simulink model "robust_tracking_integral"  (R2020b)
settings: Solver=ode45  StartTime=0.0  StopTime=5  FixedStep=T/10  RelTol=1e-3
values from neighbouring files (symbols this model uses):
  daq =     [params_inertial_case.mat]    (also in params_resonant_case.mat)
  degs2rpm = 0.166666666667    [params_inertial_case.mat]    (also in params_resonant_case.mat)
  drv =     [params_inertial_case.mat]    (also in params_resonant_case.mat)
  gbox =     [params_inertial_case.mat]    (also in params_resonant_case.mat)
  mld =     [params_inertial_case.mat]    (also in params_resonant_case.mat)
  mot =     [params_inertial_case.mat]    (also in params_resonant_case.mat)
  rads2rpm = 9.54929658551    [params_inertial_case.mat]    (also in params_resonant_case.mat)
  rpm2rads = 0.10471975512    [params_inertial_case.mat]    (also in params_resonant_case.mat)
  sens =     [params_inertial_case.mat]    (also in params_resonant_case.mat)
  tau_hat = 0.00714370660323    [params_estimated_LAB0.mat]
undefined symbols (not defined in the file or in its folder): Beq, ctrl, denH1, Jeq, k_spring, Ke, Ki, N_u, N_x, numH1, step_size
settings Model: Creator=utente  LastModifiedBy=gioel
settings DataIOCC: ReturnWorkspaceOutputs=off

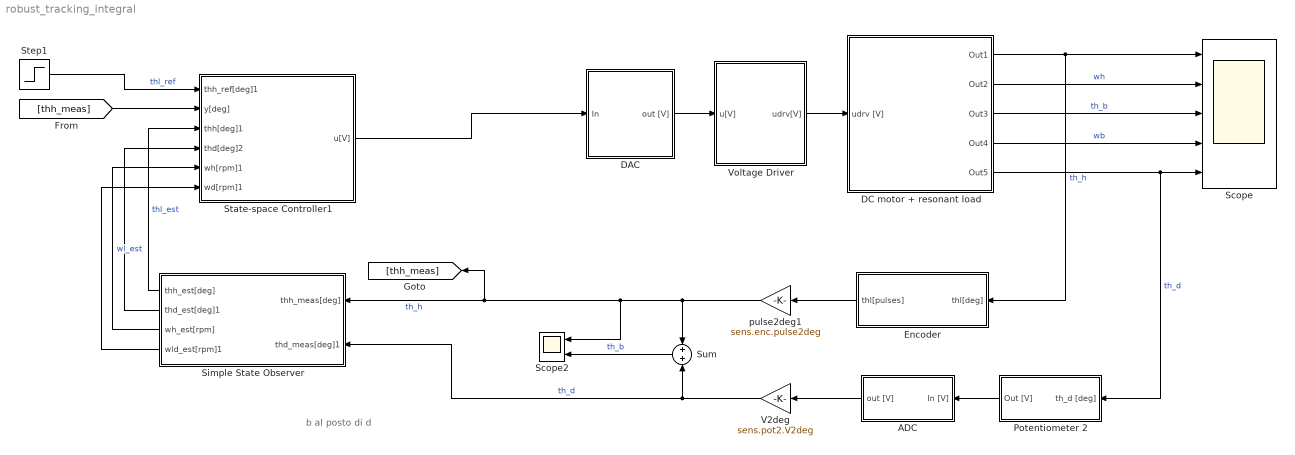
== system robust_tracking_integral ==
  note: b al posto di d
  ADC : Subsystem
  DAC : Subsystem
  DC motor + resonant load : Subsystem
  Encoder : Subsystem
  Potentiometer 2 : Subsystem
  Scope : Scope  NumInputPorts=5
  Scope2 : Scope  NumInputPorts=2
  Simple State Observer : Subsystem
  State-space Controller1 : Subsystem
  Step1 : Step  After=step_size  SampleTime=0
  Sum : Sum
  V2deg : Gain  Gain=sens.pot2.V2deg
  Voltage Driver : Subsystem
  pulse2deg1 : Gain  Gain=sens.enc.pulse2deg
  wires:
  DC motor + resonant load/3(Out3) -> Scope/3  "th_b"
  DAC/1(out [V]) -> Voltage Driver/1(u[V])
  DC motor + resonant load/2(Out2) -> Scope/2  "wh"
  DC motor + resonant load/1(Out1) -> Scope/1, Encoder/1(thl[deg])  "th_h"
  DC motor + resonant load/5(Out5) -> Scope/5, Potentiometer 2/1(th_d [deg])  "th_d"
  Encoder/1(thl[pulses]) -> pulse2deg1/1
  Voltage Driver/1(udrv[V]) -> DC motor + resonant load/1(udrv [V])
  pulse2deg1/1 -> Scope2/1, Simple State Observer/1(thh_meas[deg]), [thh_meas], Sum/1  "th_h"
  Potentiometer 2/1(Out [V]) -> ADC/1(In [V])
  V2deg/1 -> Simple State Observer/2(thd_meas[deg]1), Sum/2  "th_d"
  Sum/1 -> Scope2/2  "th_b"
  ADC/1(out [V]) -> V2deg/1
  DC motor + resonant load/4(Out4) -> Scope/4  "wb"
  Step1/1 -> State-space Controller1/1(thh_ref[deg]1)  "thl_ref"
  Simple State Observer/1(thh_est[deg]) -> State-space Controller1/3(thh[deg]1)  "thl_est"
  Simple State Observer/2(thd_est[deg]1) -> State-space Controller1/4(thd[deg]2)
  Simple State Observer/3(wh_est[rpm]) -> State-space Controller1/5(wh[rpm]1)  "wl_est"
  Simple State Observer/4(wld_est[rpm]1) -> State-space Controller1/6(wd[rpm]1)
  State-space Controller1/1(u[V]) -> DAC/1(In)
  [thh_meas] -> State-space Controller1/2(y[deg])

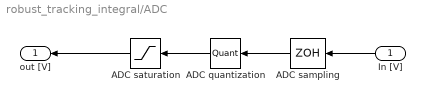
== system robust_tracking_integral/ADC ==
  In [V] : Inport
  ADC quantization : Quantizer  QuantizationInterval=daq.dac.q
  ADC saturation : Saturate  UpperLimit=daq.dac.fs  LowerLimit=-daq.dac.fs
  ADC sampling : ZeroOrderHold  SampleTime=0.001
  out [V] : Outport
  wires:
  ADC saturation/1 -> out [V]/1
  In [V]/1 -> ADC sampling/1
  ADC quantization/1 -> ADC saturation/1
  ADC sampling/1 -> ADC quantization/1

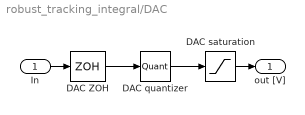
== system robust_tracking_integral/DAC ==
  In : Inport
  DAC quantizer : Quantizer  QuantizationInterval=daq.dac.q
  DAC saturation : Saturate  UpperLimit=daq.dac.fs  LowerLimit=-daq.dac.fs
  DAC ZOH : ZeroOrderHold  SampleTime=0.001
  out [V] : Outport
  wires:
  DAC ZOH/1 -> DAC quantizer/1
  DAC quantizer/1 -> DAC saturation/1
  In/1 -> DAC ZOH/1
  DAC saturation/1 -> out [V]/1

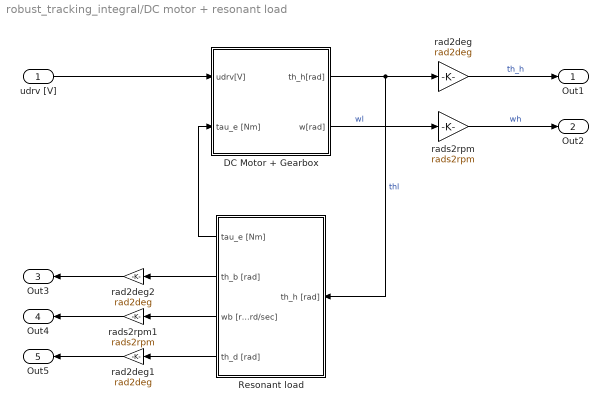
== system robust_tracking_integral/DC motor + resonant load ==
  udrv [V] : Inport
  DC Motor + Gearbox : Subsystem
  Resonant load : Subsystem
  rad2deg : Gain  Gain=rad2deg
  rad2deg1 : Gain  Gain=rad2deg
  rad2deg2 : Gain  Gain=rad2deg
  "rads2rpm " : Gain  Gain=rads2rpm
  "rads2rpm1 " : Gain  Gain=rads2rpm
  Out1 : Outport
  Out2 : Outport  Port=2
  Out3 : Outport  Port=3
  Out4 : Outport  Port=4
  Out5 : Outport  Port=5
  wires:
  Resonant load/3(wb [rard/sec]) -> "rads2rpm1 "/1
  Resonant load/4(th_d [rad]) -> rad2deg1/1
  "rads2rpm1 "/1 -> Out4/1
  rad2deg/1 -> Out1/1  "th_h"
  "rads2rpm "/1 -> Out2/1  "wh"
  rad2deg2/1 -> Out3/1
  udrv [V]/1 -> DC Motor + Gearbox/1(udrv[V])
  Resonant load/2(th_b [rad]) -> rad2deg2/1
  rad2deg1/1 -> Out5/1
  DC Motor + Gearbox/1(th_h[rad]) -> Resonant load/1(th_h [rad]), rad2deg/1  "thl"
  DC Motor + Gearbox/2(w[rad]) -> "rads2rpm "/1  "wl"
  Resonant load/1(tau_e [Nm]) -> DC Motor + Gearbox/2(tau_e [Nm])

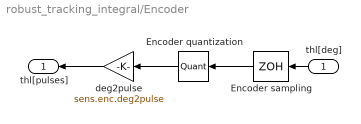
== system robust_tracking_integral/Encoder ==
  thl[deg] : Inport
  Encoder quantization : Quantizer  QuantizationInterval=sens.enc.pulse2deg
  Encoder sampling : ZeroOrderHold  SampleTime=-1
  deg2pulse : Gain  Gain=sens.enc.deg2pulse
  thl[pulses] : Outport
  wires:
  thl[deg]/1 -> Encoder sampling/1
  Encoder quantization/1 -> deg2pulse/1
  Encoder sampling/1 -> Encoder quantization/1
  deg2pulse/1 -> thl[pulses]/1

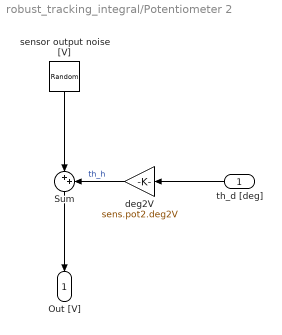
== system robust_tracking_integral/Potentiometer 2 ==
  th_d [deg] : Inport
  Sum : Sum  Inputs=|++
  deg2V : Gain  Gain=sens.pot2.deg2V
  "sensor output noise [V] " : RandomNumber  Variance=3.5e-7  SampleTime=0.1
  Out [V] : Outport
  wires:
  th_d [deg]/1 -> deg2V/1
  deg2V/1 -> Sum/2  "th_h"
  "sensor output noise [V] "/1 -> Sum/1
  Sum/1 -> Out [V]/1

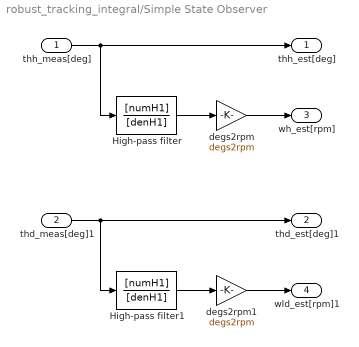
== system robust_tracking_integral/Simple State Observer ==
  thh_meas[deg] : Inport
  thd_meas[deg]1 : Inport  Port=2
  High-pass filter : TransferFcn  Numerator=[numH1]  Denominator=[denH1]
  High-pass filter1 : TransferFcn  Numerator=[numH1]  Denominator=[denH1]
  degs2rpm : Gain  Gain=degs2rpm
  degs2rpm1 : Gain  Gain=degs2rpm
  thh_est[deg] : Outport
  thd_est[deg]1 : Outport  Port=2
  wh_est[rpm] : Outport  Port=3
  wld_est[rpm]1 : Outport  Port=4
  wires:
  thh_meas[deg]/1 -> thh_est[deg]/1, High-pass filter/1
  High-pass filter/1 -> degs2rpm/1
  degs2rpm/1 -> wh_est[rpm]/1
  thd_meas[deg]1/1 -> thd_est[deg]1/1, High-pass filter1/1
  High-pass filter1/1 -> degs2rpm1/1
  degs2rpm1/1 -> wld_est[rpm]1/1

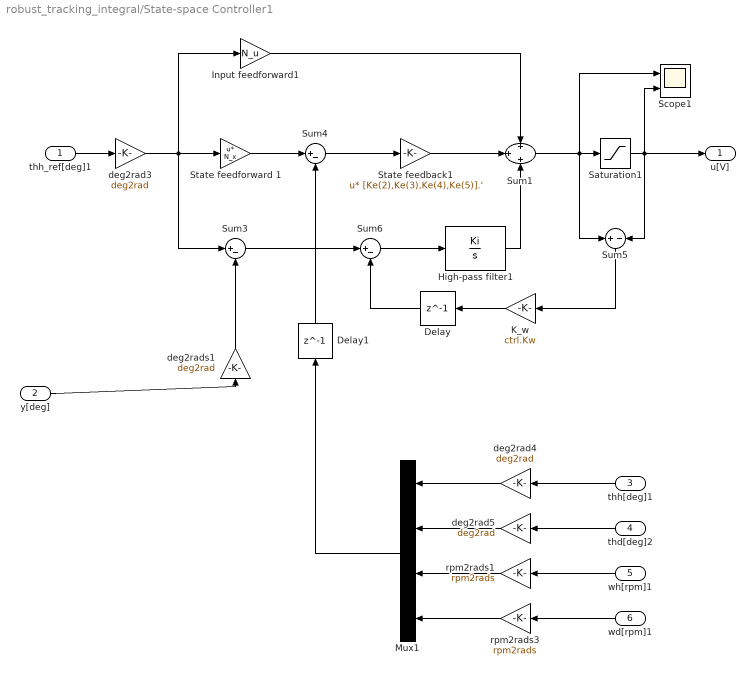
== system robust_tracking_integral/State-space Controller1 ==
  thh_ref[deg]1 : Inport
  y[deg] : Inport  Port=2
  thh[deg]1 : Inport  Port=3
  thd[deg]2 : Inport  Port=4
  wh[rpm]1 : Inport  Port=5
  wd[rpm]1 : Inport  Port=6
  Delay : Delay  DelayLength=1  InitialCondition=0
  Delay1 : Delay  DelayLength=1  InitialCondition=0
  High-pass filter1 : TransferFcn  Numerator=Ki  Denominator=[1 0]
  Input feedforward1 : Gain  Gain=N_u
  K_w : Gain  Gain=ctrl.Kw
  Mux1 : Mux
  Saturation1 : Saturate  UpperLimit=10  LowerLimit=-10
  Scope1 : Scope  NumInputPorts=2
  State feedback1 : Gain  Gain=[Ke(2),Ke(3),Ke(4),Ke(5)].'  Multiplication=Matrix(u*K)
  State feedforward	1 : Gain  Gain=N_x  Multiplication=Matrix(u*K)
  Sum1 : Sum  Inputs=+|+|+
  Sum3 : Sum  Inputs=|+-
  Sum4 : Sum  Inputs=|+-
  Sum5 : Sum  Inputs=+|-
  Sum6 : Sum  Inputs=|+-
  deg2rad3 : Gain  Gain=deg2rad
  deg2rad4 : Gain  Gain=deg2rad
  deg2rad5 : Gain  Gain=deg2rad
  deg2rads1 : Gain  Gain=deg2rad
  rpm2rads1 : Gain  Gain=rpm2rads
  rpm2rads3 : Gain  Gain=rpm2rads
  u[V] : Outport
  wires:
  Delay/1 -> Sum6/2
  Sum6/1 -> High-pass filter1/1
  deg2rads1/1 -> Sum3/2
  y[deg]/1 -> deg2rads1/1
  Sum1/1 -> Sum5/1, Scope1/1, Saturation1/1
  Delay1/1 -> Sum4/2
  K_w/1 -> Delay/1
  High-pass filter1/1 -> Sum1/3
  Sum5/1 -> K_w/1
  Sum3/1 -> Sum6/1
  State feedback1/1 -> Sum1/2
  Sum4/1 -> State feedback1/1
  deg2rad3/1 -> Sum3/1, Input feedforward1/1, State feedforward	1/1
  Saturation1/1 -> Sum5/2, Scope1/2, u[V]/1
  State feedforward	1/1 -> Sum4/1
  Input feedforward1/1 -> Sum1/1
  deg2rad5/1 -> Mux1/2
  Mux1/1 -> Delay1/1
  rpm2rads1/1 -> Mux1/3
  wd[rpm]1/1 -> rpm2rads3/1
  wh[rpm]1/1 -> rpm2rads1/1
  thh[deg]1/1 -> deg2rad4/1
  deg2rad4/1 -> Mux1/1
  thd[deg]2/1 -> deg2rad5/1
  rpm2rads3/1 -> Mux1/4
  thh_ref[deg]1/1 -> deg2rad3/1

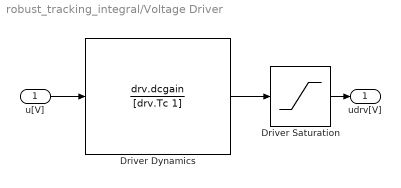
== system robust_tracking_integral/Voltage Driver ==
  u[V] : Inport
  Driver Dynamics : TransferFcn  Numerator=drv.dcgain  Denominator=[drv.Tc 1]
  Driver Saturation : Saturate  UpperLimit=12  LowerLimit=-12
  udrv[V] : Outport
  wires:
  Driver Dynamics/1 -> Driver Saturation/1
  Driver Saturation/1 -> udrv[V]/1
  u[V]/1 -> Driver Dynamics/1

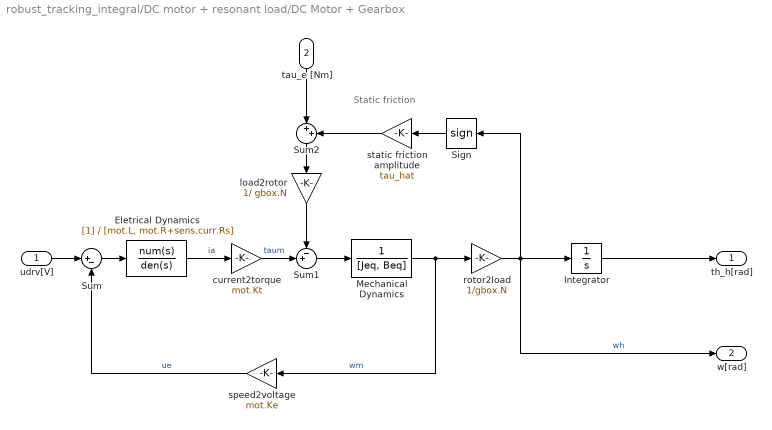
== system robust_tracking_integral/DC motor + resonant load/DC Motor + Gearbox ==
  note: Static friction
  udrv[V] : Inport
  tau_e [Nm] : Inport  Port=2
  Eletrical Dynamics : TransferFcn  Denominator=[mot.L, mot.R+sens.curr.Rs]
  Integrator : Integrator
  Mechanical Dynamics : TransferFcn  Denominator=[Jeq, Beq]
  Sign : Signum  ZeroCross=off
  Sum : Sum  Inputs=|+-
  Sum1 : Sum  Inputs=-+|
  Sum2 : Sum  Inputs=|++
  current2torque : Gain  Gain=mot.Kt
  load2rotor : Gain  Gain=1/ gbox.N
  rotor2load : Gain  Gain=1/gbox.N
  speed2voltage : Gain  Gain=mot.Ke
  static friction amplitude : Gain  Gain=tau_hat
  th_h[rad] : Outport  VectorParamsAs1DForOutWhenUnconnected=off
  w[rad] : Outport  Port=2  VectorParamsAs1DForOutWhenUnconnected=off
  wires:
  Eletrical Dynamics/1 -> current2torque/1  "ia"
  udrv[V]/1 -> Sum/1
  Sum/1 -> Eletrical Dynamics/1
  current2torque/1 -> Sum1/2  "taum"
  Sum1/1 -> Mechanical Dynamics/1
  Mechanical Dynamics/1 -> rotor2load/1, speed2voltage/1  "wm"
  rotor2load/1 -> w[rad]/1, Integrator/1, Sign/1  "wh"
  Integrator/1 -> th_h[rad]/1
  Sign/1 -> static friction amplitude/1
  speed2voltage/1 -> Sum/2  "ue"
  load2rotor/1 -> Sum1/1
  Sum2/1 -> load2rotor/1
  static friction amplitude/1 -> Sum2/2
  tau_e [Nm]/1 -> Sum2/1

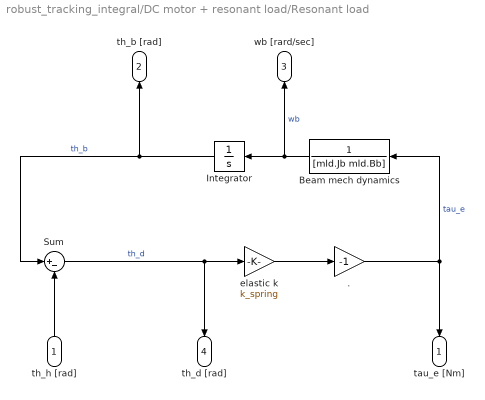
== system robust_tracking_integral/DC motor + resonant load/Resonant load ==
  th_h [rad] : Inport
  . : Gain  Gain=-1
  Beam mech dynamics : TransferFcn  Numerator=[0 1]  Denominator=[mld.Jb mld.Bb]
  Integrator : Integrator
  Sum : Sum  Inputs=|+-
  elastic k : Gain  Gain=k_spring
  tau_e [Nm] : Outport
  th_b [rad] : Outport  Port=2
  wb [rard/sec] : Outport  Port=3
  th_d [rad] : Outport  Port=4
  wires:
  th_h [rad]/1 -> Sum/2
  Sum/1 -> th_d [rad]/1, elastic k/1  "th_d"
  elastic k/1 -> ./1
  ./1 -> Beam mech dynamics/1, tau_e [Nm]/1  "tau_e"
  Beam mech dynamics/1 -> Integrator/1, wb [rard/sec]/1  "wb"
  Integrator/1 -> th_b [rad]/1, Sum/1  "th_b"
